simulink subsystem "FeaturesReferenceGenerator"  (R2020b)
settings: Solver=VariableStepAuto  StartTime=0.0  StopTime=10.0  RelTol=1e-3
model mask{C_features_0=C_features_0, C_features_desired=C_features_desired, Cdesired_T_C0=Cdesired_T_C0.double, Ts=Ts, t0=0, tf=0, no_traj=on}
  mask prompts: C_features_0 "C_features_0 (initial features in camera frame)"; C_features_desired "C_features_desired (desired features in camera frame)"; Cdesired_T_C0 "Cdesired_T_C0 (camera initial frame w.r.t. camera desired frame)"; t0 "Initial Time"; tf "Final Time"
settings Model: Creator=marco  LastModifiedBy=marco

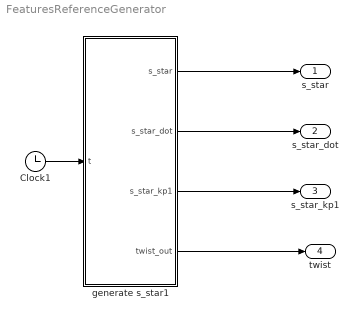
== system FeaturesReferenceGenerator ==
  Clock1 : Clock
  generate s_star1 : MATLAB Function  TreatAsAtomicUnit=on
  s_star : Outport
  s_star_dot : Outport  Port=2
  s_star_kp1 : Outport  Port=3
  twist : Outport  Port=4
  wires:
  Clock1/1 -> generate s_star1/1(t)
  generate s_star1/3(s_star_kp1) -> s_star_kp1/1
  generate s_star1/1(s_star) -> s_star/1
  generate s_star1/2(s_star_dot) -> s_star_dot/1
  generate s_star1/4(twist_out) -> twist/1

== matlab function FeaturesReferenceGenerator/generate s_star1 ==
  data: t input; s_star output; s_star_dot output; s_star_kp1 output; C_features_0 parameter double; C_features_desired parameter double; Cdesired_T_C0 parameter double; Ts parameter double; no_traj parameter boolean; twist_out output; t0 parameter; tf parameter
function [s_star,s_star_dot, s_star_kp1, twist_out] = fcn(t, C_features_0, C_features_desired, Cdesired_T_C0, Ts, no_traj, t0, tf)

if no_traj
    s_star = C_features_desired(:);
    s_star_kp1 = C_features_desired(:);
    twist_out = zeros(6,1);
    s_star_dot = zeros(size(s_star));
    return
end

% common
pos_ti = t0;
ang_ti = t0;

pos_tf = tf;
ang_tf = tf;


scalarTrajPos = @(t)quinticTraj(t,0,1,pos_ti,pos_tf);
scalarTrajQuat = @(t,deltaAng)quinticTraj(t,0,deltaAng,ang_ti,ang_tf);


t_kp1 = t + Ts;

initial_quat = [1 0 0 0];
pi = [0;0;0];

final_quat = rotm2quat(Cdesired_T_C0(1:3,1:3));
pf = Cdesired_T_C0(1:3,4);

[Qt, wt] = quatInterp(t, initial_quat, final_quat, scalarTrajQuat);
Rt = quat2rotm(Qt);
[Qt_kp1] = quatInterp(t_kp1, initial_quat, final_quat, scalarTrajQuat);
Rt_kp1 = quat2rotm(Qt_kp1);

[pt, ptdot] = positionInterp(t, pi, pf, scalarTrajPos);
[pt_kp1] = positionInterp(t_kp1, pi, pf, scalarTrajPos);

Tt = [Rt, pt; 0 0 0 1];
Tt_kp1 = [Rt_kp1, pt_kp1; 0 0 0 1];

FEATURE_star = homtrans(Tt, C_features_0);
FEATURE_star_kp1 = homtrans(Tt_kp1, C_features_0);
FEATURE_star_dot = zeros(size(FEATURE_star));
for i=1:size(C_features_0,2)
    FEATURE_star_dot(:,i) = skew(wt)*Rt*C_features_0(:,i) + ptdot(:);
%     FEATURE_star_dot(:,i) = Rt*skew(wt)*FEATURE_star(:,i) + ptdot(:);
end

twist_out = zeros(6,1);
twist_out(4:6) = -wt;
twist_out(1:3) = -(skew(pt)*wt + ptdot);
% wt_out = Rt*wt;
% ptdot_out = skew(pt)*Rt*wt + Rt*ptdot;
% wt_out = Rt'*wt;
% ptdot_out = -Rt'*skew(pt)*wt + Rt'*ptdot;

s_star = FEATURE_star(:);
s_star_kp1 = FEATURE_star_kp1(:);
s_star_dot = FEATURE_star_dot(:);
